simulink model "test"  (R2017b)
settings: Solver=VariableStepAuto  StartTime=0.0  StopTime=10.0  RelTol=1e-3
settings Model: Creator=guozhenglong  LastModifiedBy=guozhenglong

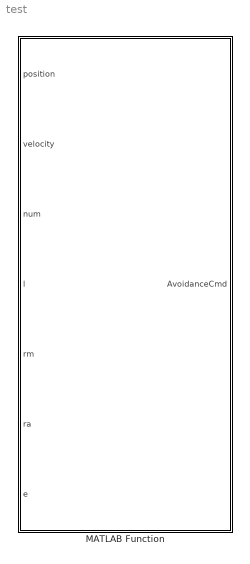
== system test ==
  MATLAB Function : MATLAB Function  TreatAsAtomicUnit=on

== matlab function test/MATLAB Function ==
  data: position input; AvoidanceCmd output; velocity input; num input; l input; rm input; ra input; e input
function AvoidanceCmd = getAvoidanceCmd(position, velocity,num,l,rm,ra,e)
% position velocity: 3xn
%   此处显示详细说明
    distans = cell(num,num);
    cmd_all = zeros(3,num);
    for i =1:num
        for j=1:num
           dis = zeros(3,1);
           for k =1:3
               dis(k,1) = (position(k,i)-position(k,j))+l*(velocity(k,i)-velocity(k,j));
           end
           distans{i,j}= dis;
        end
        k=1;
        cmd_i =  zeros(3,1);
        while(k<=num)
            if(i~=k)
                cmd_i = cmd_i + avoidCmd(distans{i,k}, rm,ra,e); % 3x1
            end
            k= k+1;
        end
        cmd_all(:,i) = cmd_i;
    end
    AvoidanceCmd = cmd_all;
end
